simulink model "sim2_control_Architectures"  (R2021a)
settings: Solver=VariableStepAuto  StartTime=0.0  StopTime=10  RelTol=1e-3
undefined symbols (not defined in the file or in its folder): a, b, kd2, kd3, ki3, kp1, kp2, kp3
settings Model: Creator=sokserey  LastModifiedBy=sokserey

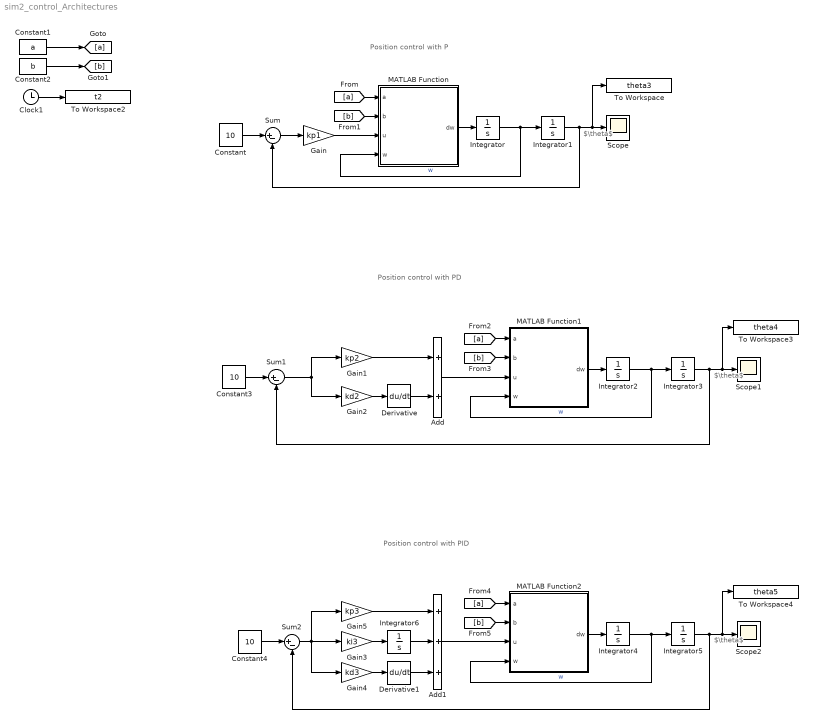
== system sim2_control_Architectures ==
  note: Position control with PID
  note: $\theta$
  note: $\theta$
  note: Position control with P
  note: Position control with PD
  note: $\theta$
  Add : Sum
  Add1 : Sum  Inputs=+++
  Clock1 : Clock
  Constant : Constant  Value=10
  Constant1 : Constant  Value=a
  Constant2 : Constant  Value=b
  Constant3 : Constant  Value=10
  Constant4 : Constant  Value=10
  Derivative : Derivative
  Derivative1 : Derivative
  Gain : Gain  Gain=kp1
  Gain1 : Gain  Gain=kp2
  Gain2 : Gain  Gain=kd2
  Gain3 : Gain  Gain=ki3
  Gain4 : Gain  Gain=kd3
  Gain5 : Gain  Gain=kp3
  Integrator{,1..6} (7 alike) : Integrator
  MATLAB Function : MATLAB Function  TreatAsAtomicUnit=on
  MATLAB Function1 : MATLAB Function  TreatAsAtomicUnit=on
  MATLAB Function2 : MATLAB Function  TreatAsAtomicUnit=on
  Scope : Scope
  Scope1 : Scope
  Scope2 : Scope
  Sum : Sum  Inputs=|+-
  Sum1 : Sum  Inputs=|+-
  Sum2 : Sum  Inputs=|+-
  To Workspace : ToWorkspace  VariableName=theta3  SampleTime=-1
      settings: Save2DSignal=2-D array (concatenate along first dimension)
  To Workspace2 : ToWorkspace  VariableName=t2  SampleTime=-1
      settings: Save2DSignal=2-D array (concatenate along first dimension)
  To Workspace3 : ToWorkspace  VariableName=theta4  SampleTime=-1
      settings: Save2DSignal=2-D array (concatenate along first dimension)
  To Workspace4 : ToWorkspace  VariableName=theta5  SampleTime=-1
      settings: Save2DSignal=2-D array (concatenate along first dimension)
  wires:
  Constant4/1 -> Sum2/1
  Derivative/1 -> Add/2
  Add/1 -> MATLAB Function1/3(u)
  MATLAB Function2/1(dw) -> Integrator4/1
  Constant3/1 -> Sum1/1
  Gain1/1 -> Add/1
  Gain2/1 -> Derivative/1
  [a] -> MATLAB Function2/1(a)
  Integrator6/1 -> Add1/2
  Sum2/1 -> Gain4/1, Gain5/1, Gain3/1
  MATLAB Function/1(dw) -> Integrator/1
  Sum/1 -> Gain/1
  Gain/1 -> MATLAB Function/3(u)
  Integrator3/1 -> To Workspace3/1, Scope1/1, Sum1/2
  Integrator5/1 -> Sum2/2, Scope2/1, To Workspace4/1
  [b] -> MATLAB Function2/2(b)
  Gain3/1 -> Integrator6/1
  Gain5/1 -> Add1/1
  [a] -> MATLAB Function/1(a)
  Derivative1/1 -> Add1/3
  Integrator1/1 -> Sum/2, To Workspace/1, Scope/1
  [b] -> MATLAB Function1/2(b)
  Gain4/1 -> Derivative1/1
  Add1/1 -> MATLAB Function2/3(u)
  Sum1/1 -> Gain2/1, Gain1/1
  [b] -> MATLAB Function/2(b)
  Integrator/1 -> Integrator1/1, MATLAB Function/4(w)  "w"
  Constant/1 -> Sum/1
  Constant1/1 -> [a]
  Integrator2/1 -> MATLAB Function1/4(w), Integrator3/1  "w"
  Integrator4/1 -> Integrator5/1, MATLAB Function2/4(w)  "w"
  MATLAB Function1/1(dw) -> Integrator2/1
  Constant2/1 -> [b]
  Clock1/1 -> To Workspace2/1
  [a] -> MATLAB Function1/1(a)

== matlab function sim2_control_Architectures/MATLAB Function ==
  data: a input; dw output; b input; u input; w input
function dw = fcn(a,b,u,w)

dw = -a*w+b*u;

== matlab function sim2_control_Architectures/MATLAB Function1 ==
  data: a input; dw output; b input; u input; w input
function dw = fcn(a,b,u,w)

dw = -a*w+b*u;

== matlab function sim2_control_Architectures/MATLAB Function2 ==
  data: a input; dw output; b input; u input; w input
function dw = fcn(a,b,u,w)

dw = -a*w+b*u;
